simulink model "Continuous_Time_Design"  (R2024b)
settings: Solver=FixedStepAuto  StartTime=0.0  StopTime=10  FixedStep=0.01  RelTol=1e-3
libraries: slpidlib x3, simulink x1
(part 4 of 4)

== matlab function Continuous_Time_Design/MOTORLARA VERİLECEK DATA1 ==
  data: F input; F_M output
function F_M = fcn(F)
F1 = F(1);
F2 = F(2);
F3 = F(3);
F4 = F(4);
F5 = F(5);
F6 = F(6);

if F1 == 0
    F1 = -F2;
elseif F2 == 0
    F2 = -F1;
end

if F3 == 0
    F3 = -F4;
elseif F4 == 0
    F4 = -F3;
end

if F5 == 0
    F5 = -F6;
elseif F6 == 0
    F6 = -F5;
end

F_M = [F1; F2; F3; F4; F5; F6];

end

== matlab function Continuous_Time_Design/MOTORLARA VERİLECEK DATA ==
  data: F input; F_M output
function F_M = fcn(F)
F1 = F(1);
F2 = F(2);
F3 = F(3);
F4 = F(4);
F5 = F(5);
F6 = F(6);

if F1 == 0
    F1 = -F2;
elseif F2 == 0
    F2 = -F1;
end

if F3 == 0
    F3 = -F4;
elseif F4 == 0
    F4 = -F3;
end

if F5 == 0
    F5 = -F6;
elseif F6 == 0
    F6 = -F5;
end

F_M = [F1; F2; F3; F4; F5; F6];

end

== matlab function Continuous_Time_Design/MATLAB Function ==
  data: t1 input; x_p output; t2 input; t3 input; y_p output
function [x_p, y_p] = fcn(t1, t2, t3)

x_p = 10*cos(t1) + 9*cos(t1+t2) + 5.7*cos(t1+t2+t3);
y_p = 10*sin(t1) + 9*sin(t1+t2) + 5.7*sin(t1+t2+t3);

end

== matlab function Continuous_Time_Design/FEEDBACK LİNEARIZATION1 ==
  data: d2q_des1 input; F output; d2q_des2 input; d2q_des3 input; states input; T output
function [F, T] = fcn(d2q_des1, d2q_des2, d2q_des3, states)

theta1 = states(1);
theta2 = states(2);
theta3 = states(3);
D_THETA_1 = states(4);
D_THETA_2 = states(5);
D_THETA_3 = states(6);

% Tork Tendon Matrisi
a11 =  -0.00500000000000000 ;
a12 =  0.00500000000000000 ;
A = [a11 a12];


%A = [a11 a12 a13 a14 a15 a16; a21 a22 a23 a24 a25 a26; a31 a32 a33 a34 a35 a36];

T1 =  -0.00018*D_THETA_1*D_THETA_2*sin(theta2) - 3.42e-5*D_THETA_1*D_THETA_2*sin(theta2 + theta3) - 3.078e-5*D_THETA_1*D_THETA_3*sin(theta3) - 3.42e-5*D_THETA_1*D_THETA_3*sin(theta2 + theta3) - 9.0e-5*(D_THETA_2^2)*sin(theta2) - 1.71e-5*(D_THETA_2^2)*sin(theta2 + theta3) - 3.078e-5*D_THETA_2*D_THETA_3*sin(theta3) - 3.42e-5*D_THETA_2*D_THETA_3*sin(theta2 + theta3) - 1.539e-5*(D_THETA_3^2)*sin(theta3) - 1.71e-5*(D_THETA_3^2)*sin(theta2 + theta3) + d2q_des1*(0.00018*cos(theta2) + 3.078e-5*cos(theta3) + 3.42e-5*cos(theta2 + theta3) + 0.000296104833333333) + d2q_des2*(9.0e-5*cos(theta2) + 3.078e-5*cos(theta3) + 1.71e-5*cos(theta2 + theta3) + 9.77715e-5) + d2q_des3*(1.539e-5*cos(theta3) + 1.71e-5*cos(theta2 + theta3) + 1.13715e-5) + 0.018639*cos(theta1) + 0.008829*cos(theta1 + theta2) + 0.00167751*cos(theta1 + theta2 + theta3) ;
T2 =  9.0e-5*(D_THETA_1^2)*sin(theta2) + 1.71e-5*(D_THETA_1^2)*sin(theta2 + theta3) - 3.078e-5*D_THETA_1*D_THETA_3*sin(theta3) - 3.078e-5*D_THETA_2*D_THETA_3*sin(theta3) - 1.539e-5*(D_THETA_3^2)*sin(theta3) + d2q_des1*(9.0e-5*cos(theta2) + 3.078e-5*cos(theta3) + 1.71e-5*cos(theta2 + theta3) + 9.77715e-5) + d2q_des2*(3.078e-5*cos(theta3) + 9.77715e-5) + d2q_des3*(1.539e-5*cos(theta3) + 1.13715e-5) + 0.008829*cos(theta1 + theta2) + 0.00167751*cos(theta1 + theta2 + theta3) ;
T3 =  1.539e-5*(D_THETA_1^2)*sin(theta3) + 1.71e-5*(D_THETA_1^2)*sin(theta2 + theta3) + 3.078e-5*D_THETA_1*D_THETA_2*sin(theta3) + 1.539e-5*(D_THETA_2^2)*sin(theta3) + d2q_des1*(1.539e-5*cos(theta3) + 1.71e-5*cos(theta2 + theta3) + 1.13715e-5) + d2q_des2*(1.539e-5*cos(theta3) + 1.13715e-5) + 1.13715e-5*d2q_des3 + 0.00167751*cos(theta1 + theta2 + theta3) ;

T = [T1; T2; T3];

%inv_A = transpose(A)/((A*transpose(A)));
%F_1 = inv_A*T1;
%F_2 = inv_A*T2;
%F_3 = inv_A*T3;

F_1 = lsqnonneg(A, T1);
F_2 = lsqnonneg(A, T2);
F_3 = lsqnonneg(A, T3);

F = [F_1; F_2; F_3];
%F = F + [0.01; 0.01; 0.01; 0.01; 0.01; 0.01];

== matlab function Continuous_Time_Design/FEEDBACK LİNEARIZATION2 ==
  data: d2q_des1 input; F output; d2q_des2 input; d2q_des3 input; states input; T output
function [F, T] = fcn(d2q_des1, d2q_des2, d2q_des3, states)

theta1 = states(1);
theta2 = states(2);
theta3 = states(3);
D_THETA_1 = states(4);
D_THETA_2 = states(5);
D_THETA_3 = states(6);


T1 =  -0.00018*D_THETA_1*D_THETA_2*sin(theta2) - 3.42e-5*D_THETA_1*D_THETA_2*sin(theta2 + theta3) - 3.078e-5*D_THETA_1*D_THETA_3*sin(theta3) - 3.42e-5*D_THETA_1*D_THETA_3*sin(theta2 + theta3) - 9.0e-5*(D_THETA_2^2)*sin(theta2) - 1.71e-5*(D_THETA_2^2)*sin(theta2 + theta3) - 3.078e-5*D_THETA_2*D_THETA_3*sin(theta3) - 3.42e-5*D_THETA_2*D_THETA_3*sin(theta2 + theta3) - 1.539e-5*(D_THETA_3^2)*sin(theta3) - 1.71e-5*(D_THETA_3^2)*sin(theta2 + theta3) + d2q_des1*(0.00018*cos(theta2) + 3.078e-5*cos(theta3) + 3.42e-5*cos(theta2 + theta3) + 0.000296104833333333) + d2q_des2*(9.0e-5*cos(theta2) + 3.078e-5*cos(theta3) + 1.71e-5*cos(theta2 + theta3) + 9.77715e-5) + d2q_des3*(1.539e-5*cos(theta3) + 1.71e-5*cos(theta2 + theta3) + 1.13715e-5) + 0.018639*cos(theta1) + 0.008829*cos(theta1 + theta2) + 0.00167751*cos(theta1 + theta2 + theta3) ;
T2 =  9.0e-5*(D_THETA_1^2)*sin(theta2) + 1.71e-5*(D_THETA_1^2)*sin(theta2 + theta3) - 3.078e-5*D_THETA_1*D_THETA_3*sin(theta3) - 3.078e-5*D_THETA_2*D_THETA_3*sin(theta3) - 1.539e-5*(D_THETA_3^2)*sin(theta3) + d2q_des1*(9.0e-5*cos(theta2) + 3.078e-5*cos(theta3) + 1.71e-5*cos(theta2 + theta3) + 9.77715e-5) + d2q_des2*(3.078e-5*cos(theta3) + 9.77715e-5) + d2q_des3*(1.539e-5*cos(theta3) + 1.13715e-5) + 0.008829*cos(theta1 + theta2) + 0.00167751*cos(theta1 + theta2 + theta3) ;
T3 =  1.539e-5*(D_THETA_1^2)*sin(theta3) + 1.71e-5*(D_THETA_1^2)*sin(theta2 + theta3) + 3.078e-5*D_THETA_1*D_THETA_2*sin(theta3) + 1.539e-5*(D_THETA_2^2)*sin(theta3) + d2q_des1*(1.539e-5*cos(theta3) + 1.71e-5*cos(theta2 + theta3) + 1.13715e-5) + d2q_des2*(1.539e-5*cos(theta3) + 1.13715e-5) + 1.13715e-5*d2q_des3 + 0.00167751*cos(theta1 + theta2 + theta3) ;

T = [T1; T2; T3];


if T1<0
    F1 = T1/-0.005;
    F2 = 0;
else
    F1 = 0;
    F2 = T2/-0.005;
end

if T2<0
    F3 = T2/-0.005;
    F4 = 0;
else
    F3 = 0;
    F4 = T2/-0.005;
end

if T3<0
    F5 = 0;
    F6 = T3/-0.005;
else
    F5 = T3/0.005;
    F6 = 0;
end

F = [F1; F2; F3; F4; F5; F6];

end

== matlab function Continuous_Time_Design/İMPEDANS KONTROL2/MATLAB Function ==
  data: qe1 input; u1 output; dqe1 input; d2qe1 input; u2 output; u3 output; qe2 input; dqe2 input; d2qe2 input; qe3 input; dqe3 input; d2qe3 input
function [u1, u2, u3] = fcn(qe1, dqe1, d2qe1, qe2, dqe2, d2qe2, qe3, dqe3, d2qe3)

u1 = 0.1*d2qe1 + 10*dqe1 + 10*qe1 ;
u2 = 0.09*d2qe2 + 9*dqe2 + 9*qe2 ;
u3 = 0.057*d2qe3 + 5.7*dqe3 + 5.7*qe3 ;
end
